simulink model "hdlFrame_Blur_3D_MLFB"  (R2022b)
settings: Solver=VariableStepAuto  StartTime=0.0  StopTime=0.0  RelTol=1e-3
libraries: visionsources x1
settings Model: Creator=quangha  LastModifiedBy=quangha
settings OptimizationCC: BlockReduction=off  ConditionallyExecuteInputs=off  DefaultParameterBehavior=Inlined
settings DebuggingCC: AlgebraicLoopMsg=error
settings HardwareCC: ProdBitPerPointer=32  ProdBitPerSizeT=32  ProdBitPerPtrDiffT=32  ProdLargestAtomicFloat=None  ProdIntDivRoundTo=Undefined  ProdEndianess=Unspecified  ProdWordSize=32  ProdHWDeviceType=ASIC/FPGA->ASIC/FPGA  TargetBitPerPointer=64  TargetBitPerSizeT=64  TargetBitPerPtrDiffT=64  TargetLongLongMode=on  TargetIntDivRoundTo=Zero  TargetEndianess=LittleEndian  TargetWordSize=64  TargetHWDeviceType=Custom Processor->MATLAB Host Computer  ProdEqTarget=off
settings RTWCC: PlatformDefinition=Embedded Code

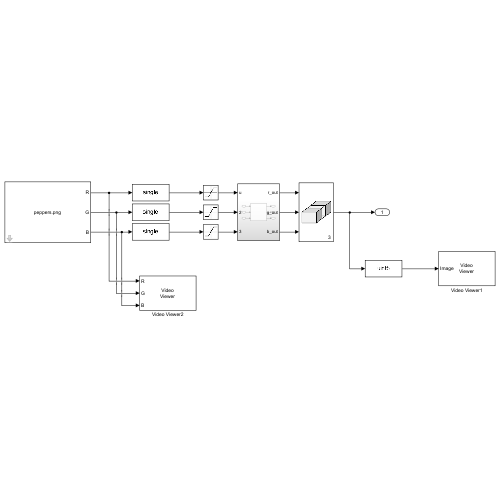
[thumbnail: Simulink's stored preview of the top-level diagram]
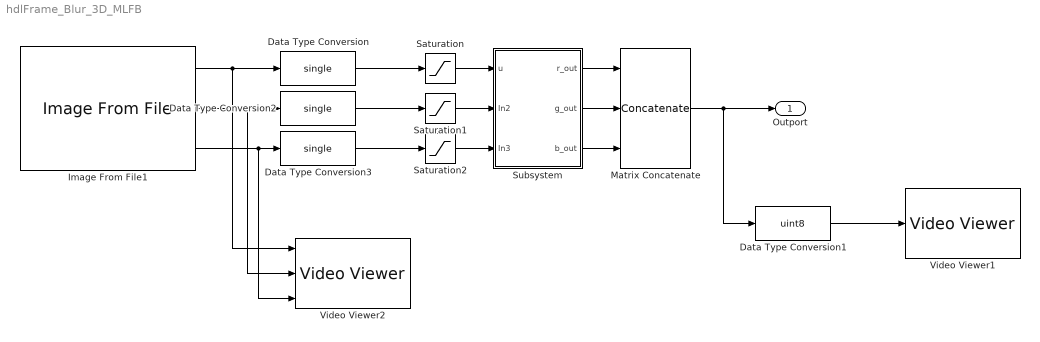
== system hdlFrame_Blur_3D_MLFB ==
  Data Type Conversion : DataTypeConversion  OutDataTypeStr=single  SaturateOnIntegerOverflow=off  RndMeth=Floor
  Data Type Conversion1 : DataTypeConversion  OutDataTypeStr=uint8  SaturateOnIntegerOverflow=off  RndMeth=Floor
  Data Type Conversion2 : DataTypeConversion  OutDataTypeStr=single  SaturateOnIntegerOverflow=off  RndMeth=Floor
  Data Type Conversion3 : DataTypeConversion  OutDataTypeStr=single  SaturateOnIntegerOverflow=off  RndMeth=Floor
  Image From File1 : visionsources/Image From File  Tag=vipblks_nd  FileName=peppers.png  Ts=0.1  imagePorts=Separate color signals  OutPortLabels=R|G|B  ImageDataType=Inherit from input image  sdImageDataType=uint(8)  Signed=on  WordLength=16  FractionLengthMode=User-defined  FractionLength=15
  Matrix Concatenate : Concatenate  NumInputs=3  Mode=Multidimensional array  ConcatenateDimension=3
  Saturation : Saturate  UpperLimit=255  LowerLimit=1
  Saturation1 : Saturate  UpperLimit=255  LowerLimit=1
  Saturation2 : Saturate  UpperLimit=255  LowerLimit=1
  Subsystem : Subsystem
  Video Viewer1 : VideoViewer  FigPos=[1331.66666666667 929.333333333333 418 304]
  Video Viewer2 : VideoViewer  imagePorts=separate color signals  FigPos=[918.333333333333 926.666666666667 412 301.333333333333]
  Outport : Outport
  wires:
  Data Type Conversion/1 -> Saturation/1
  Saturation/1 -> Subsystem/1(u)
  Data Type Conversion1/1 -> Video Viewer1/1
  Image From File1/1 -> Video Viewer2/1, Data Type Conversion/1
  Image From File1/2 -> Video Viewer2/2, Data Type Conversion2/1
  Image From File1/3 -> Video Viewer2/3, Data Type Conversion3/1
  Data Type Conversion3/1 -> Saturation2/1
  Data Type Conversion2/1 -> Saturation1/1
  Saturation1/1 -> Subsystem/2(In2)
  Saturation2/1 -> Subsystem/3(In3)
  Subsystem/1(r_out) -> Matrix Concatenate/1
  Subsystem/2(g_out) -> Matrix Concatenate/2
  Subsystem/3(b_out) -> Matrix Concatenate/3
  Matrix Concatenate/1 -> Data Type Conversion1/1, Outport/1

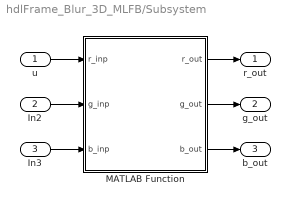
== system hdlFrame_Blur_3D_MLFB/Subsystem ==
  u : Inport
  In2 : Inport  Port=2
  In3 : Inport  Port=3
  MATLAB Function : MATLAB Function  TreatAsAtomicUnit=on
  r_out : Outport
  g_out : Outport  Port=2
  b_out : Outport  Port=3
  wires:
  u/1 -> MATLAB Function/1(r_inp)
  MATLAB Function/1(r_out) -> r_out/1
  In2/1 -> MATLAB Function/2(g_inp)
  In3/1 -> MATLAB Function/3(b_inp)
  MATLAB Function/2(g_out) -> g_out/1
  MATLAB Function/3(b_out) -> b_out/1

== matlab function hdlFrame_Blur_3D_MLFB/Subsystem/MATLAB Function ==
  data: r_inp input; r_out output; g_inp input; b_inp input; g_out output; b_out output
function [r_out, g_out, b_out] = image_blurring(r_inp, g_inp, b_inp)
r_out = hdl.npufun(@blurring_kernel, [4, 4], r_inp);
g_out = hdl.npufun(@blurring_kernel, [4, 4], g_inp);
b_out = hdl.npufun(@blurring_kernel, [4, 4], b_inp);
end

function out = blurring_kernel(in)
hN = single(...
    [0.0608    0.0625    0.0625    0.0608;
     0.0625    0.0642    0.0642    0.0625;
     0.0625    0.0642    0.0642    0.0625;
     0.0608    0.0625    0.0625    0.0608]);
out = sum(in(:).*hN(:), 'native');
end
